simulink model "LQR"  (R2016b)
settings: Solver=FixedStepAuto  StartTime=0.0  StopTime=stoptime  FixedStep=stepsize  RelTol=1e-3
values from neighbouring files (symbols this model uses):
  A = [0.2 0.7 ... (first row only)    [main.m]
  B = [0.1 0.5]'    [main.m]
  m = 1    [main.m]
  n = 2    [main.m]
  xm = [cos(th(i)) sin(th(i))]'    [main.m]    (also in runMPC.m = x0+dist)
settings Model: Creator=Berk  LastModifiedBy=Berk

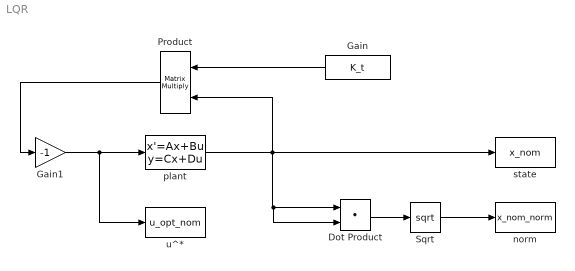
== system LQR ==
  Dot Product : DotProduct  InputSameDT=on  OutDataTypeStr=Inherit: Inherit via internal rule
  Gain : FromWorkspace  VariableName=K_t  SampleTime=0
  Gain1 : Gain  Gain=-1
  Product : Product  Multiplication=Matrix(*)
  Sqrt : Sqrt  SaturateOnIntegerOverflow=on
  norm : ToWorkspace  VariableName=x_nom_norm  SaveFormat=Timeseries  SampleTime=-1
  plant : StateSpace  A=A  B=B  C=eye(n)  D=zeros(n,m)  X0=xm
  state : ToWorkspace  VariableName=x_nom  SaveFormat=Timeseries  SampleTime=-1
  u^* : ToWorkspace  VariableName=u_opt_nom  SaveFormat=Timeseries  SampleTime=-1
  wires:
  plant/1 -> Dot Product/2, Dot Product/1, Product/2, state/1
  Gain1/1 -> u^*/1, plant/1
  Product/1 -> Gain1/1
  Gain/1 -> Product/1
  Dot Product/1 -> Sqrt/1
  Sqrt/1 -> norm/1
